simulink model "FAM_lab_scale_turbine_generator"  (R2023b)
settings: Solver=VariableStepAuto  StartTime=0.0  StopTime=120  FixedStep=0.002  MaxStep=0.01  RelTol=1e-3  EnableMultiTasking=on
libraries: FAM_lab_scale x1, turbine_generator x1
settings Model: DataDictionary=FAM_parameters_lab_scale.sldd  ExtModeTrigDuration=10000  Creator=cmmcguir  LastModifiedBy=cmmcguir
settings SolverCC: AlgebraicLoopSolver=TrustRegion  PositivePriorityOrder=on
settings DataIOCC: ReturnWorkspaceOutputs=off
settings OptimizationCC: LifeSpan=inf
settings DebuggingCC: UnconnectedInputMsg=warning  UnconnectedOutputMsg=warning  UnconnectedLineMsg=warning  ArithmeticOperatorsInVariantConditions=warning
settings ModelReferenceCC: EnableRefExpFcnMdlSchedulingChecks=on
settings SFSimCC: SimUseLocalCustomCode=off  CustomCodeUndefinedFunction=UseInterfaceOnly
settings RTWCC: Description=QUARC Win64 Target  SystemTargetFile=quarc_win64.tlc  TemplateMakefile=quarc_default_tmf  RTWUseLocalCustomCode=off
settings CodeAppCC: StateflowObjectComments=on
settings STFCustomTargetCC: TargetPreCompLibLocation=C:\PROGRA~3\QUARC\lib\2023b\win64\release  ConcurrentExecutionCompliant=on  GRTInterface=on  SystemTargetFile=quarc_win64.tlc
settings GRTTargetCC: TargetPreCompLibLocation=C:\PROGRA~3\QUARC\lib\2023b\win64\release  ParMdlRefBuildCompliant=off  CompOptLevelCompliant=off  CombineOutputUpdateFcns=off  MatFileLogging=off  CPPClassGenCompliant=off  GRTInterface=on  UseToolchainInfoCompliant=off  ExtMode=on  ExtModeMexFile=quarc_comm
settings ConfigComp: CovMetricSettings=dswe
settings SimscapeCC: SimscapeLogType=all  SimscapeLogLimitData=off

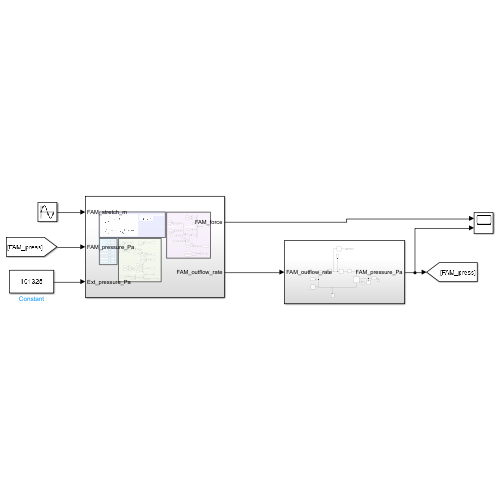
[thumbnail: Simulink's stored preview of the top-level diagram]
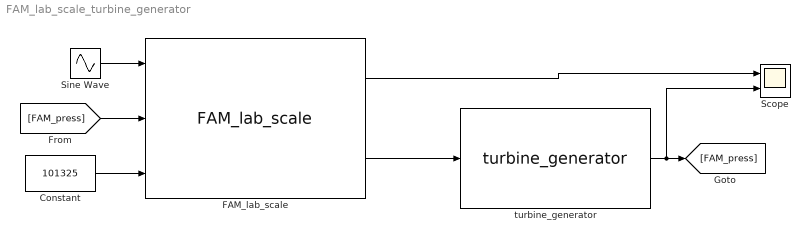
== system FAM_lab_scale_turbine_generator ==
  Constant : Constant  Value=101325
  FAM_lab_scale : FAM_lab_scale/FAM_lab_scale  SystemSampleTime=-1  VariantActivationTime=update diagram  AllowFlexibleInterface=on  Latency=0  AutoFrameSizeCalculation=off
  Scope : Scope  NumInputPorts=2
  Sine Wave : Sin  Amplitude=0.01  SampleTime=0
  turbine_generator : turbine_generator/turbine_generator  SystemSampleTime=-1  VariantActivationTime=update diagram  AllowFlexibleInterface=on  Latency=0  AutoFrameSizeCalculation=off
  wires:
  FAM_lab_scale/2 -> turbine_generator/1
  Constant/1 -> FAM_lab_scale/3
  turbine_generator/1 -> Scope/2, [FAM_press]
  [FAM_press] -> FAM_lab_scale/2
  Sine Wave/1 -> FAM_lab_scale/1
  FAM_lab_scale/1 -> Scope/1
